simulink model "steamjacket"  (R2020b)
settings: Solver=VariableStepAuto  StartTime=0.0  StopTime=10.0  RelTol=1e-3
settings Model: Creator=Adam  LastModifiedBy=Adam

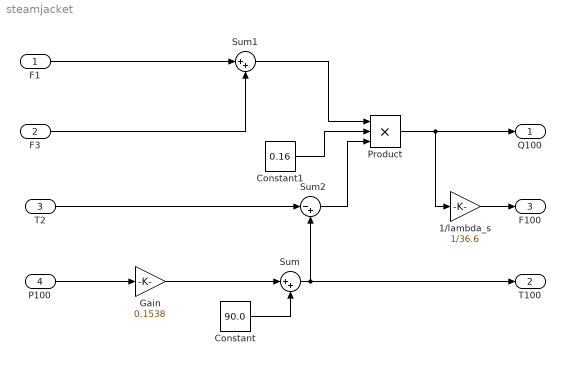
== system steamjacket ==
  F1 : Inport
  F3 : Inport  Port=2
  T2 : Inport  Port=3
  P100 : Inport  Port=4
  1/lambda_s : Gain  Gain=1/36.6
  Constant : Constant  Value=90.0
  Constant1 : Constant  Value=0.16
  Gain : Gain  Gain=0.1538
  Product : Product  Inputs=3
  Sum : Sum  Inputs=|++
  Sum1 : Sum  Inputs=|++
  Sum2 : Sum  Inputs=|-+
  Q100 : Outport
  T100 : Outport  Port=2
  F100 : Outport  Port=3
  wires:
  Constant/1 -> Sum/2
  P100/1 -> Gain/1
  Gain/1 -> Sum/1
  Sum/1 -> T100/1, Sum2/2
  F1/1 -> Sum1/1
  F3/1 -> Sum1/2
  T2/1 -> Sum2/1
  Sum1/1 -> Product/1
  Constant1/1 -> Product/2
  Sum2/1 -> Product/3
  Product/1 -> 1/lambda_s/1, Q100/1
  1/lambda_s/1 -> F100/1
